simulink model "discrete_linear"  (R2017a)
settings: Solver=VariableStepAuto  StartTime=0.0  StopTime=10.0  RelTol=1e-3
undefined symbols (not defined in the file or in its folder): DCd, NCd, T
settings Model: Creator=julio  LastModifiedBy=julio

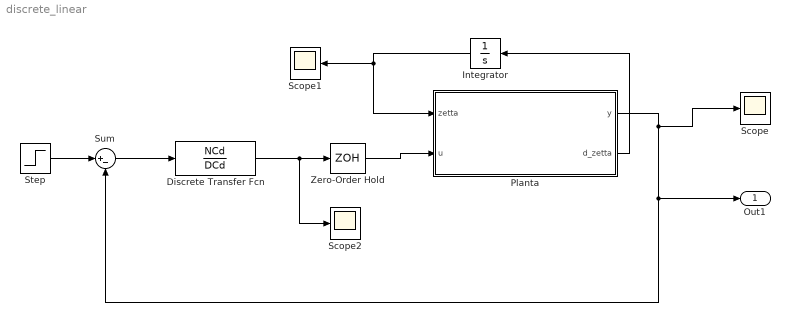
== system discrete_linear ==
  Discrete Transfer Fcn : DiscreteTransferFcn  Numerator=NCd  Denominator=DCd  SampleTime=T  a0EqualsOne=on
  Integrator : Integrator
  Planta : MATLAB Function  TreatAsAtomicUnit=on  RTWFcnName=linear_func  RTWFileName=linear_func
      settings: MinAlgLoopOccurrences=on  RTWFileNameOpts=User specified
  Scope : Scope
  Scope1 : Scope
  Scope2 : Scope
  Step : Step  Time=0  After=0.3  SampleTime=0
  Sum : Sum  Inputs=|+-
  Zero-Order Hold : ZeroOrderHold  SampleTime=-1
  Out1 : Outport  SignalName=y
  wires:
  Zero-Order Hold/1 -> Planta/2(u)
  Sum/1 -> Discrete Transfer Fcn/1
  Integrator/1 -> Planta/1(zetta), Scope1/1
  Discrete Transfer Fcn/1 -> Scope2/1, Zero-Order Hold/1
  Planta/1(y) -> Scope/1, Out1/1, Sum/2
  Planta/2(d_zetta) -> Integrator/1
  Step/1 -> Sum/1

== matlab function discrete_linear/Planta ==
  data: zetta input size=4; u input size=1; y output size=1; d_zetta output size=4
function [ y, d_zetta] = linear_func( zetta, u )
%LINEAR_FUNC Summary of this function goes here
%   Detailed explanation goes here
    MJ = 1.0731; % [kg]
    m  = 0.209;  % [kg]
    l  = 0.3302; % [m]
    bK = 5.4;    % [N.s/(m²)]
    Kr = 1.0717; % [N/V]
    g  = 9.81;   % [m/s²]
    
    A = [0 1 0 0
        0 -bK/MJ m*g/MJ 0
        0 0 0 1
        0 bK/(MJ*l) -((g/l)+(m*g/(MJ*l))) 0];
    
    B = [0 
        Kr/MJ
        0
        -Kr/(MJ*l)];
    
    C = [1 0 0 0];
    
    D = [0];
    
    d_zetta = A*zetta + B*u;
    
    y = C*zetta + D*u;
end
